simulink model "Simulation"  (R2021b)
settings: Solver=VariableStepAuto  StartTime=0.0  StopTime=10.0  RelTol=1e-3
undefined symbols (not defined in the file): A, B, K, l, n
settings Model: Creator=mluser  LastModifiedBy=mluser

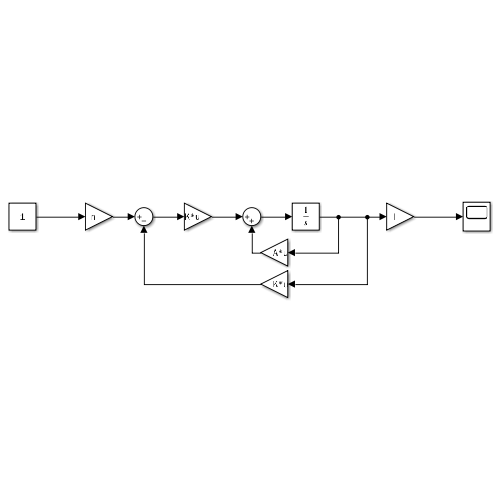
[thumbnail: Simulink's stored preview of the top-level diagram]
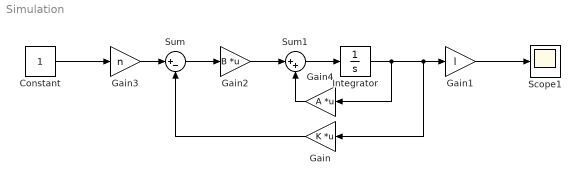
== system Simulation ==
  Constant : Constant
  Gain : Gain  Gain=K  Multiplication=Matrix(K*u)
  Gain1 : Gain  Gain=l
  Gain2 : Gain  Gain=B  Multiplication=Matrix(K*u)
  Gain3 : Gain  Gain=n
  Gain4 : Gain  Gain=A  Multiplication=Matrix(K*u)
  Integrator : Integrator
  Scope1 : Scope
  Sum : Sum  Inputs=|+-
  Sum1 : Sum  Inputs=|++
  wires:
  Sum/1 -> Gain2/1
  Gain/1 -> Sum/2
  Integrator/1 -> Gain4/1, Gain1/1, Gain/1
  Gain2/1 -> Sum1/1
  Sum1/1 -> Integrator/1
  Gain4/1 -> Sum1/2
  Gain1/1 -> Scope1/1
  Constant/1 -> Gain3/1
  Gain3/1 -> Sum/1
